simulink model "stugverter_monitor"  (R2026a)
settings: Solver=FixedStepDiscrete  StopTime=inf  FixedStep=0.01
undefined symbols (not defined in the file): calibration_modulation, calibration_request, control_enable_request, control_fault_reset, control_mode_request, g_calibration_complete, g_calibration_sample_count, g_duty_u, g_duty_v, g_duty_w, g_foc_exec_time_us, g_foc_isr_counter, g_gate_drivers_enabled, g_hil_mode_enable, g_meas_curr_u, g_meas_curr_v, g_meas_curr_w, g_meas_speed, g_meas_theta_mech, g_spd_ref_rpm, g_supervisor_active_mode, g_supervisor_pwm_enable, Hardware_100Hz, HW, open_loop_electrical_hz, open_loop_modulation, torque_ref_nm
libraries: xcpprotocollib x4
settings Model: Creator=probst  LastModifiedBy=probst

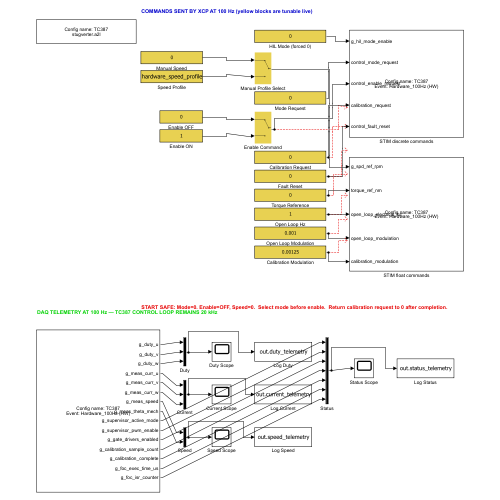
[thumbnail: Simulink's stored preview of the top-level diagram]
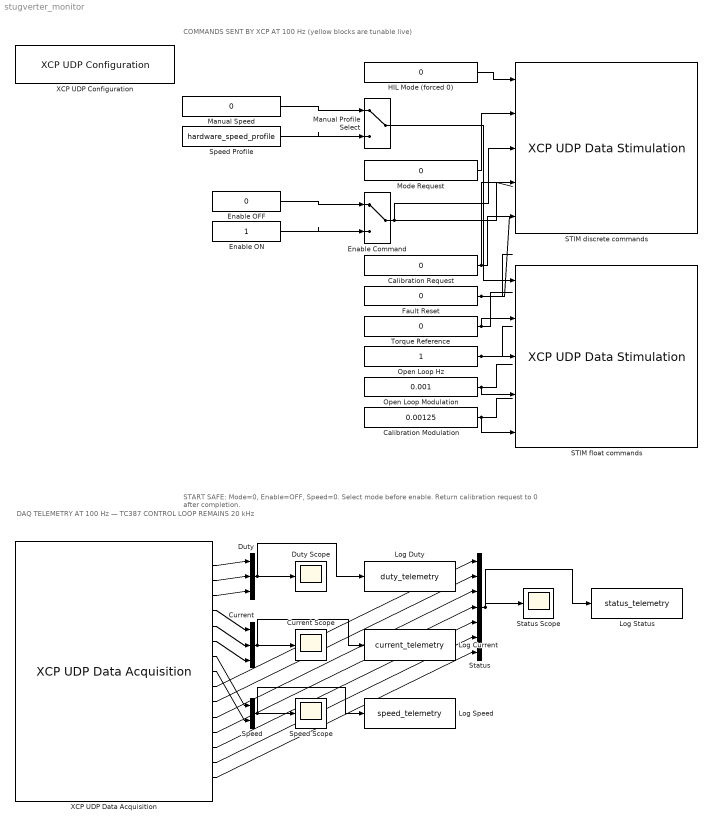
== system stugverter_monitor ==
  note: COMMANDS SENT BY XCP AT 100 Hz (yellow blocks are tunable live)
  note: DAQ TELEMETRY AT 100 Hz — TC387 CONTROL LOOP REMAINS 20 kHz
  note: START SAFE: Mode=0, Enable=OFF, Speed=0. Select mode before enable. Return calibration request to 0 after completion.
  Calibration Modulation : Constant  Value=0.00125  OutDataTypeStr=double  SampleTime=0.01
  Calibration Request : Constant  Value=0  OutDataTypeStr=double  SampleTime=0.01
  Current : Mux  Inputs=3
  Current Scope : Scope
  Duty : Mux  Inputs=3
  Duty Scope : Scope
  Enable Command : ManualSwitch
  Enable OFF : Constant  Value=0  OutDataTypeStr=double  SampleTime=0.01
  Enable ON : Constant  OutDataTypeStr=double  SampleTime=0.01
  Fault Reset : Constant  Value=0  OutDataTypeStr=double  SampleTime=0.01
  HIL Mode (forced 0) : Constant  Value=0  OutDataTypeStr=double  SampleTime=0.01
  Log Current : ToWorkspace  VariableName=current_telemetry  SaveFormat=Timeseries  SampleTime=-1
  Log Duty : ToWorkspace  VariableName=duty_telemetry  SaveFormat=Timeseries  SampleTime=-1
  Log Speed : ToWorkspace  VariableName=speed_telemetry  SaveFormat=Timeseries  SampleTime=-1
  Log Status : ToWorkspace  VariableName=status_telemetry  SaveFormat=Timeseries  SampleTime=-1
  Manual Profile Select : ManualSwitch
  Manual Speed : Constant  Value=0  OutDataTypeStr=double  SampleTime=0.01
  Mode Request : Constant  Value=0  OutDataTypeStr=double  SampleTime=0.01
  Open Loop Hz : Constant  OutDataTypeStr=double  SampleTime=0.01
  Open Loop Modulation : Constant  Value=0.001  OutDataTypeStr=double  SampleTime=0.01
  STIM discrete commands : xcpprotocollib/UDP/XCP UDP Data Stimulation  SlaveName=TC387  A2LFile=C:\Users\probst\Desktop\stugverter\firmware\stugverter.a2l  EventName=Hardware_100Hz (HW)  SelectedMeasurements=g_hil_mode_enable;control_mode_request;control_enable_request;calibration_request;control_fault_reset  EnableTimestamp=off  InputOrOutputDatatype=Raw values as double (no Compu method conversion)
      settings: LibrarySourceBlock=vntxcplib/UDP/XCP UDP Data Stimulation
  STIM float commands : xcpprotocollib/UDP/XCP UDP Data Stimulation  SlaveName=TC387  A2LFile=C:\Users\probst\Desktop\stugverter\firmware\stugverter.a2l  EventName=Hardware_100Hz (HW)  SelectedMeasurements=g_spd_ref_rpm;torque_ref_nm;open_loop_electrical_hz;open_loop_modulation;calibration_modulation  EnableTimestamp=off  InputOrOutputDatatype=Raw values as double (no Compu method conversion)
      settings: LibrarySourceBlock=vntxcplib/UDP/XCP UDP Data Stimulation
  Speed : Mux  Inputs=2
  Speed Profile : FromWorkspace  VariableName=hardware_speed_profile  SampleTime=0.01
  Speed Scope : Scope
  Status : Mux  Inputs=7
  Status Scope : Scope
  Torque Reference : Constant  Value=0  OutDataTypeStr=double  SampleTime=0.01
  XCP UDP Configuration : xcpprotocollib/UDP/XCP UDP Configuration  Priority=-100  SlaveName=TC387  SlaveID=1  A2LFile=C:\Users\probst\Desktop\stugverter\firmware\stugverter.a2l  EnableSecurity=off  ConnectMode=off  EnableStatus=off  SampleTime=0.01  HeaderErrDet=on  CTRScheme=One counter for all CTOs and DTOs  LocalAddress=192.168.0.100  LocalPort=auto  DAQTimeout=Inf
      settings: LibrarySourceBlock=vntxcplib/UDP/XCP UDP Configuration
  XCP UDP Data Acquisition : xcpprotocollib/UDP/XCP UDP Data Acquisition  SlaveName=TC387  A2LFile=C:\Users\probst\Desktop\stugverter\firmware\stugverter.a2l  EventName=Hardware_100Hz (HW)  SelectedMeasurements=g_duty_u;g_duty_v;g_duty_w;g_meas_curr_u;g_meas_curr_v;g_meas_curr_w;g_meas_speed;g_meas_theta_mech;g_supervisor_active_mode;g_supervisor_pwm_enable;g_gate_drivers_enabled;g_calibration_sample_count;g_calibration_complete;g_foc_exec_time_us;g_foc_isr_counter  DAQPriority=0  SampleTime=0.01  EnableTimestamp=off  InputOrOutputDatatype=Raw values as double (no Compu method conversion)
      settings: LibrarySourceBlock=vntxcplib/UDP/XCP UDP Data Acquisition
  wires:
  Manual Speed/1 -> Manual Profile Select/1
  Speed Profile/1 -> Manual Profile Select/2
  Enable OFF/1 -> Enable Command/1
  Enable ON/1 -> Enable Command/2
  Duty/1 -> Duty Scope/1, Log Duty/1
  Current/1 -> Current Scope/1, Log Current/1
  Speed/1 -> Speed Scope/1, Log Speed/1
  Status/1 -> Status Scope/1, Log Status/1
  XCP UDP Data Acquisition/1 -> Duty/1
  XCP UDP Data Acquisition/2 -> Duty/2
  XCP UDP Data Acquisition/3 -> Duty/3
  XCP UDP Data Acquisition/4 -> Current/1
  XCP UDP Data Acquisition/5 -> Current/2
  XCP UDP Data Acquisition/6 -> Current/3
  XCP UDP Data Acquisition/7 -> Speed/1
  XCP UDP Data Acquisition/8 -> Speed/2
  XCP UDP Data Acquisition/9 -> Status/1
  XCP UDP Data Acquisition/10 -> Status/2
  XCP UDP Data Acquisition/11 -> Status/3
  XCP UDP Data Acquisition/12 -> Status/4
  XCP UDP Data Acquisition/13 -> Status/5
  XCP UDP Data Acquisition/14 -> Status/6
  XCP UDP Data Acquisition/15 -> Status/7
  Manual Profile Select/1 -> STIM float commands/1
  Mode Request/1 -> STIM discrete commands/2
  Enable Command/1 -> STIM discrete commands/3
  Calibration Request/1 -> STIM discrete commands/4
  Fault Reset/1 -> STIM discrete commands/5
  Torque Reference/1 -> STIM float commands/2
  Open Loop Hz/1 -> STIM float commands/3
  Open Loop Modulation/1 -> STIM float commands/4
  Calibration Modulation/1 -> STIM float commands/5
  HIL Mode (forced 0)/1 -> STIM discrete commands/1
